simulink model "go"  (R2017b)
settings: Solver=VariableStepAuto  StartTime=0.0  StopTime=10.0  RelTol=1e-3
settings Model: Creator=Administrator  LastModifiedBy=Administrator

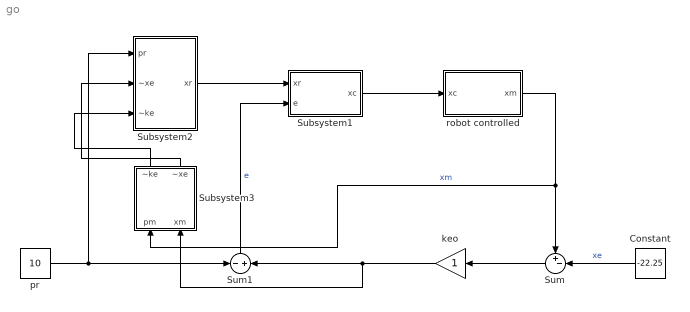
== system go ==
  Constant : Constant  Value=-22.25
  Subsystem1 : Subsystem
  Subsystem2 : Subsystem
  Subsystem3 : Subsystem
  Sum : Sum  Inputs=+-|
  Sum1 : Sum  Inputs=-|+
  keo : Gain
  pr : Constant  Value=10
  robot controlled : Subsystem
  wires:
  Constant/1 -> Sum/2  "xe"
  robot controlled/1("xm ") -> Subsystem3/1(pm), Sum/1  "xm"
  Subsystem1/1(xc) -> robot controlled/1(xc)
  Sum/1 -> keo/1
  Sum1/1 -> Subsystem1/2(e)  "e"
  keo/1 -> Subsystem3/2(xm), Sum1/2
  Subsystem2/1(xr) -> Subsystem1/1(xr)
  pr/1 -> Subsystem2/1(pr), Sum1/1
  Subsystem3/1(~ke) -> Subsystem2/3(~ke)
  Subsystem3/2(~xe) -> Subsystem2/2(~xe)

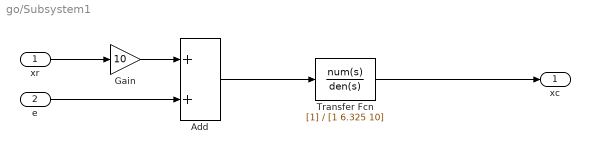
== system go/Subsystem1 ==
  xr : Inport
  e : Inport  Port=2
  Add : Sum
  Gain : Gain  Gain=10
  Transfer Fcn : TransferFcn  Denominator=[1 6.325 10]
  xc : Outport
  wires:
  xr/1 -> Gain/1
  Gain/1 -> Add/1
  e/1 -> Add/2
  Add/1 -> Transfer Fcn/1
  Transfer Fcn/1 -> xc/1

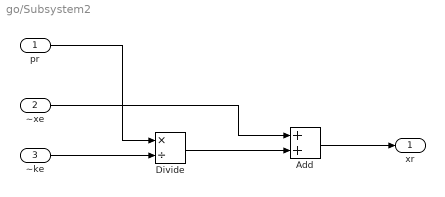
== system go/Subsystem2 ==
  pr : Inport
  ~xe : Inport  Port=2
  ~ke : Inport  Port=3
  Add : Sum
  Divide : Product  Inputs=*/
  xr : Outport
  wires:
  pr/1 -> Divide/1
  ~ke/1 -> Divide/2
  ~xe/1 -> Add/1
  Divide/1 -> Add/2
  Add/1 -> xr/1

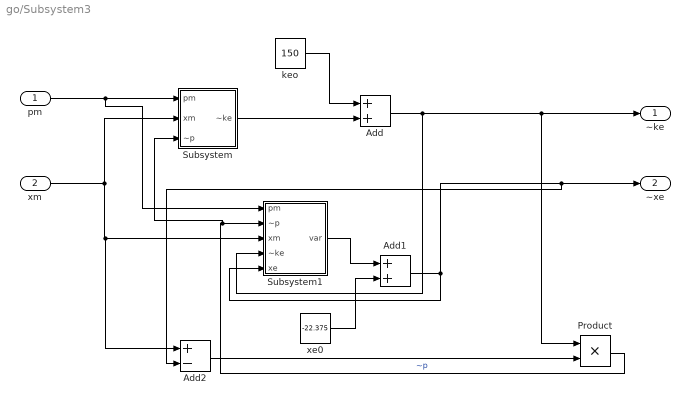
== system go/Subsystem3 ==
  pm : Inport
  xm : Inport  Port=2
  Add : Sum
  Add1 : Sum
  Add2 : Sum  Inputs=+-
  Product : Product
  Subsystem : Subsystem
  Subsystem1 : Subsystem
  keo : Constant  Value=150
  xe0 : Constant  Value=-22.375
  ~ke : Outport
  ~xe : Outport  Port=2
  wires:
  pm/1 -> Subsystem1/1(pm), Subsystem/1(pm)
  xm/1 -> Subsystem/2(xm), Add2/1, Subsystem1/3(xm)
  keo/1 -> Add/1
  Add/1 -> Subsystem1/4(~ke), Product/1, ~ke/1
  Subsystem/1(~ke) -> Add/2
  Subsystem1/1(var) -> Add1/1
  xe0/1 -> Add1/2
  Add1/1 -> Subsystem1/5("xe "), Add2/2, ~xe/1
  Add2/1 -> Product/2
  Product/1 -> Subsystem/3(~p), Subsystem1/2(~p)  "~p"

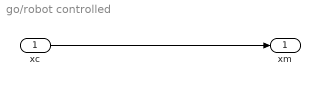
== system go/robot controlled ==
  xc : Inport
  "xm " : Outport
  wires:
  xc/1 -> "xm "/1

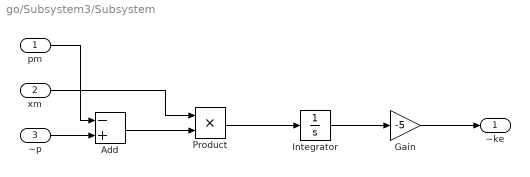
== system go/Subsystem3/Subsystem ==
  pm : Inport
  xm : Inport  Port=2
  ~p : Inport  Port=3
  Add : Sum  Inputs=-+
  Gain : Gain  Gain=-5
  Integrator : Integrator
  Product : Product
  ~ke : Outport
  wires:
  ~p/1 -> Add/2
  pm/1 -> Add/1
  xm/1 -> Product/1
  Add/1 -> Product/2
  Product/1 -> Integrator/1
  Integrator/1 -> Gain/1
  Gain/1 -> ~ke/1

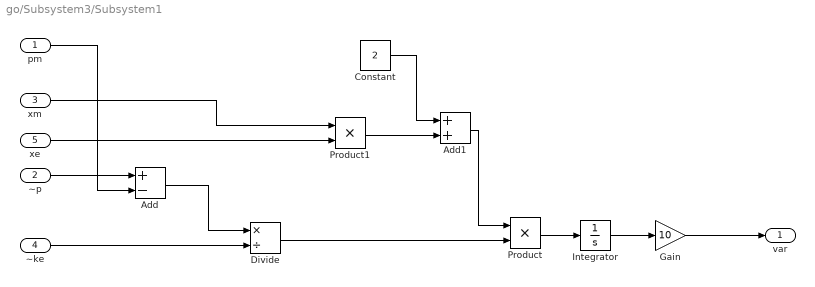
== system go/Subsystem3/Subsystem1 ==
  pm : Inport
  ~p : Inport  Port=2
  xm : Inport  Port=3
  ~ke : Inport  Port=4
  "xe " : Inport  Port=5
  Add : Sum  Inputs=+-
  Add1 : Sum
  Constant : Constant  Value=2
  Divide : Product  Inputs=*/
  Gain : Gain  Gain=10
  Integrator : Integrator
  Product : Product
  Product1 : Product
  var : Outport
  wires:
  pm/1 -> Add/2
  ~p/1 -> Add/1
  Add/1 -> Divide/1
  ~ke/1 -> Divide/2
  Divide/1 -> Product/2
  xm/1 -> Product1/1
  Constant/1 -> Add1/1
  Product1/1 -> Add1/2
  Add1/1 -> Product/1
  Integrator/1 -> Gain/1
  Gain/1 -> var/1
  "xe "/1 -> Product1/2
  Product/1 -> Integrator/1
